simulink model "flexcan_can_fd_master_s32k14"  (R2017a)
settings: Solver=FixedStepDiscrete  StartTime=0.0  StopTime=10.0  FixedStep=0.1  RelTol=1e-3  EnableMultiTasking=on
InitFcn:
  | mbd_s32k14_consistency_checks(bdroot(gcs));
undefined symbols (not defined in the file): B8, C7, D1, D2, G2, PTC6, PTC7, PTD16, PTE4, PTE5, raw_temp
libraries: mbd_s32k14_ec_toolbox x10, etargetslib x1, simulink x1
Description:
  | This model tests FlexCAN communication using CAN with Flexible Data-Rate.
  | The FlexCAN Master sends on each step a message with ID 0x3FF to the slave.
  | On each Tx Complete event Blue LED (PTD0) is toggled.
  | 
  | HW prerequisite:
  | - S32K144EVB-Q100
  | - Make sure that J107 has pin 1 and 2 connected and external power supply is provieded through J16.
  | 
  | Validation:
  | - The CAN Baudrate is set to 500 Kb/s
  | - Any CAN analizer (USB to CAN device) can be used to observe CAN traffic via board CAN port J13.
settings Model: Creator=agrigorev  LastModifiedBy=Siddharth
settings DataIOCC: ExternalInput=off  InitialState=off  LimitDataPoints=on  SaveFormat=Array  SaveOutput=off  SignalLogging=off  SaveTime=off
settings OptimizationCC: DefaultParameterBehavior=Inlined  PassReuseOutputArgsAs=Individual arguments
settings DebuggingCC: UnderspecifiedInitializationDetection=Classic  MergeDetectMultiDrivingBlocksExec=none  SolverPrmCheckMsg=warning  InheritedTsInSrcMsg=none  SingleTaskRateTransMsg=error  ParameterTunabilityLossMsg=error  UnconnectedInputMsg=error  UnconnectedOutputMsg=error  UnconnectedLineMsg=error  AllowSymbolicDim=off  UnknownTsInhSupMsg=error  StateNameClashWarn=warning  SFUnexpectedBacktrackingDiag=warning  SFNoUnconditionalDefaultTransitionDiag=warning  SFExecutionAtInitializationDiag=none
settings HardwareCC: ProdBitPerPointer=32  ProdBitPerSizeT=32  ProdBitPerPtrDiffT=32  ProdLargestAtomicInteger=Long  ProdLargestAtomicFloat=Double  ProdWordSize=32  ProdHWDeviceType=ARM Compatible->ARM Cortex
settings ModelReferenceCC: PropagateSignalLabelsOutOfModel=off
settings SFSimCC: MATLABDynamicMemAlloc=off
settings RTWCC: SystemTargetFile=mbd_s32k14.tlc  MakeCommand=mbd_s32k14_make_rtw COPY_MDLREF_INCLUDES=0  TemplateMakefile=mbd_s32k14.tmf  Description=Model Based Design Toolbox S32K14x Code Generation Target  GenerateReport=on  IncludeHyperlinkInReport=on  LaunchReport=on  GenerateTraceInfo=on  GenerateTraceReport=on  GenerateTraceReportSl=on  GenerateTraceReportSf=on  GenerateTraceReportEml=on
settings CodeAppCC: ForceParamTrailComments=on  IgnoreCustomStorageClasses=off  OperatorAnnotations=on  SimulinkDataObjDesc=on  SFDataObjDesc=on  MATLABFcnDesc=on  InsertBlockDesc=on  MATLABSourceComments=on
settings STFCustomTargetCC: MultiwordLength=256  CombineOutputUpdateFcns=on  ERTCustomFileBanners=on  SupportContinuousTime=off  SupportNonInlinedSFcns=off  RemoveResetFunc=on  MATLABClassNameForMDSCustomization=Simulink.SoftwareTarget.ERTCustomization  GRTInterface=off  SystemTargetFile=mbd_s32k14.tlc
settings ERTTargetCC: ParMdlRefBuildCompliant=off  CompOptLevelCompliant=off  ConcurrentExecutionCompliant=off  ERTFirstTimeCompliant=off  ModelStepFunctionPrototypeControlCompliant=off  CPPClassGenCompliant=off  UseToolchainInfoCompliant=off  InlinedParameterPlacement=NonHierarchical  ERTCustomFileTemplate=example_file_process.tlc
settings ConfigComp: CovMetricSettings=dw  CovHtmlReporting=on  CovSaveCumulativeToWorkspaceVar=on  CovSaveSingleToWorkspaceVar=on  CovExternalEMLEnable=off

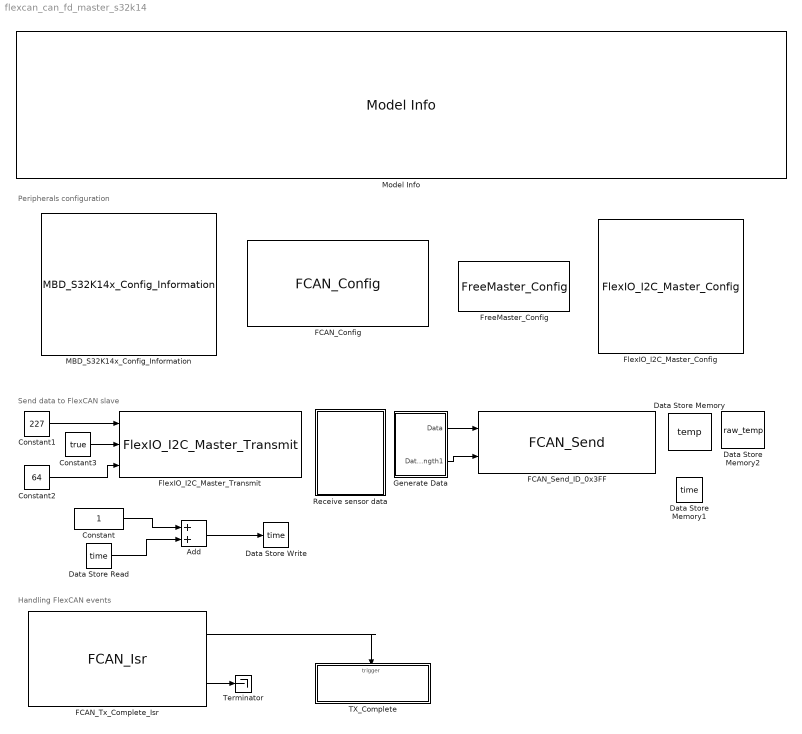
== system flexcan_can_fd_master_s32k14 ==
  note: Peripherals configuration
  note: Handling FlexCAN events
  note: Send data to FlexCAN slave
  Add : Sum  AccumDataTypeStr=uint32  OutDataTypeStr=uint32
  Constant : Constant  OutDataTypeStr=uint32
  Constant1 : Constant  Value=227  OutDataTypeStr=uint8
  Constant2 : Constant  Value=64  OutDataTypeStr=uint8
  Constant3 : Constant  Value=true
  Data Store Memory : DataStoreMemory  DataStoreName=temp  ReadBeforeWriteMsg=warning  WriteAfterWriteMsg=warning  WriteAfterReadMsg=warning  ShowAdditionalParam=off
  Data Store Memory1 : DataStoreMemory  DataStoreName=time  ReadBeforeWriteMsg=warning  WriteAfterWriteMsg=warning  WriteAfterReadMsg=warning  ShowAdditionalParam=off  OutDataTypeStr=uint32
  Data Store Memory2 : DataStoreMemory  DataStoreName=raw_temp  ReadBeforeWriteMsg=warning  WriteAfterWriteMsg=warning  WriteAfterReadMsg=warning  InitialValue=[0 0]  ShowAdditionalParam=off  OutDataTypeStr=uint8  Dimensions=2
  Data Store Read : DataStoreRead  DataStoreName=time
  Data Store Write : DataStoreWrite  DataStoreName=time
  FCAN_Config : mbd_s32k14_ec_toolbox/S32K14x/Communication Blocks/Flex CAN Blocks/FCAN_Config  Priority=1  can_instance=0  can_mode=Normal mode  can_max_num_mb=16  can_rx=PTE4 : [9] : [6] : [D1]  can_tx=PTE5 : [8] : [5] : [D2]  show_adv_opts=on  can_clk_src=Peripheral clock  can_presdiv=9  can_rjw=0  can_pseg1=3  can_pseg2=3  can_propseg=6  can_cbt_presdiv=9  can_cbt_rjw=0  can_cbt_pseg1=3  can_cbt_pseg2=3  can_cbt_propseg=6  can_fd_enable=on  can_payload=8  can_rxfifo_enable=off  can_fifo_id_filter_extended=off  can_fifo_id_filter_remote=off  can_num_id_filters=8  can_fifo_id_format=A  can_fifo_id_filter={'0x0', '0x0', '0x0', '0x0', '0x0', '0x0', '0x0', '0x0'}  can_pn_enable=off  can_wakeup_match=off  can_wakeup_timeout=off  can_timeout_en=off  can_match_timeout=1  can_multiple_matches_en=off  can_num_matches=1  can_idfilter_extendedid=off  can_idfilter_remoteframe=off  can_idfilter_type=Match exact  can_idfilter_id1=0  can_idfilter_id2=0  can_payloadfilter_enable=off  can_payloadfilter_dlclow=0  can_payloadfilter_dlchigh=0  can_payloadfilter_type=Match exact  can_payloadfilter_payload1_b0=0  can_payloadfilter_payload1_b1=0  can_payloadfilter_payload1_b2=0  can_payloadfilter_payload1_b3=0  can_payloadfilter_payload1_b4=0  can_payloadfilter_payload1_b5=0  can_payloadfilter_payload1_b6=0  can_payloadfilter_payload1_b7=0  can_payloadfilter_payload2_b0=0  can_payloadfilter_payload2_b1=0  can_payloadfilter_payload2_b2=0  can_payloadfilter_payload2_b3=0  can_payloadfilter_payload2_b4=0  can_payloadfilter_payload2_b5=0  can_payloadfilter_payload2_b6=0  can_payloadfilter_payload2_b7=0
  FCAN_Send_ID_0x3FF : mbd_s32k14_ec_toolbox/S32K14x/Communication Blocks/Flex CAN Blocks/FCAN_Send  Priority=2  can_instance=0  can_mode=Non-blocking  can_timeout_ms=0  can_mb_idx=15  can_extended_id=off  can_is_remote=off  can_id=3FF  show_adv_opts=on  can_fd_enable=on  can_enable_brs=off  can_fd_padding=0
  FCAN_Tx_Complete_Isr : mbd_s32k14_ec_toolbox/S32K14x/Communication Blocks/Flex CAN Blocks/FCAN_Isr  can_instance=0  can_event=Tx Complete
  "FlexIO_I2C_Master_Config " : mbd_s32k14_ec_toolbox/S32K14x/Communication Blocks/FlexIO Blocks /FlexIO I2C Blocks/FlexIO_I2C_Master_Config   InstanceNumber=0  DriverType=Polling  BaudRate=400000  SDA_pin=[PTD0] FXIO_D0  SCL_pin=[PTD1] FXIO_D1
  FlexIO_I2C_Master_Transmit : mbd_s32k14_ec_toolbox/S32K14x/Communication Blocks/FlexIO Blocks /FlexIO I2C Blocks/FlexIO_I2C_Master_Transmit  InstanceNumber=0  Timeout=10
  FreeMaster_Config : mbd_s32k14_ec_toolbox/S32K14x/Utility Blocks/FreeMaster_Config  interface=UART1  baudrate=57600  rxd=PTC6 : [81] : [52] : [C7]  txd=PTC7 : [80] : [51] : [B8]  mode=Poll-driven  isr_prio=15  show_adv_opts=off  use_scope=on  max_scope_vars=8  use_recorder=on  max_rec_vars=8  rec_buff_size=1024  rec_timebase=0 seconds  comm_buffer_size_auto=on  comm_buffer_size=255  comm_rqueue_size_default=on  comm_rqueue_size=32
  Generate Data : Subsystem
  MBD_S32K14x_Config_Information : mbd_s32k14_ec_toolbox/S32K14x/MBD_S32K14x_Config_Information  disp_str=|  config_params=[]
      | Target : S32K144-64KB_SRAM
      | Package : 100-pin
      | System clock : 80 MHz
      | XTAL clock : External 8 MHz
      | Compiler : GCC
      | Target Type : FLASH
      | Download Code after build : (OpenSDA: F)
      | Step Tick Interrupt Priority : 15
  Model Info : simulink/Model-Wide Utilities/Model Info  Frame=off  DisplayStringWithTags=|  HorizontalTextAlignment=Left  LeftAlignmentValue=0.02  SourceBlockDiagram=flexcan_can_fd_master_s32k14  TagMaxNumber=20
      | Model Name: %<ModelName>
      | 
      | Description: %<Description>
  Receive sensor data : Subsystem
  TX_Complete : Subsystem  TreatAsAtomicUnit=on
      settings: RTWSystemCode=Nonreusable function
  Terminator : Terminator
  wires:
  FCAN_Tx_Complete_Isr/2 -> Terminator/1
  Generate Data/2(Data Length1) -> FCAN_Send_ID_0x3FF/2
  Generate Data/1(Data) -> FCAN_Send_ID_0x3FF/1
  FCAN_Tx_Complete_Isr/1 -> TX_Complete/Trigger
  Constant2/1 -> FlexIO_I2C_Master_Transmit/3
  Constant1/1 -> FlexIO_I2C_Master_Transmit/1
  Constant3/1 -> FlexIO_I2C_Master_Transmit/2
  Constant/1 -> Add/1
  Data Store Read/1 -> Add/2
  Add/1 -> Data Store Write/1

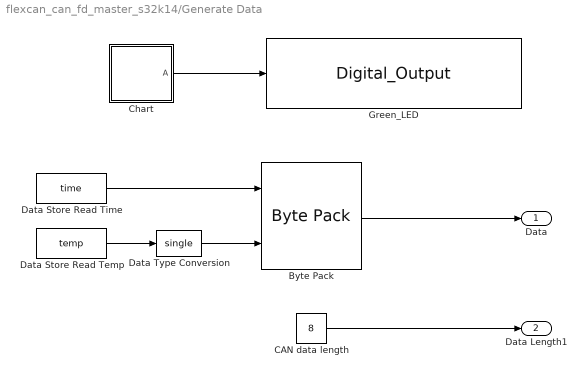
== system flexcan_can_fd_master_s32k14/Generate Data ==
  Byte Pack : etargetslib/Byte Pack  datatypes={'uint32','single'}  byteAlign=1
  CAN data length : Constant  Value=8  OutDataTypeStr=uint8
  Chart : Stateflow chart  TreatAsAtomicUnit=on
  Data Store Read Temp : DataStoreRead  DataStoreName=temp
  Data Store Read Time : DataStoreRead  DataStoreName=time
  Data Type Conversion : DataTypeConversion  OutDataTypeStr=single
  Green_LED : mbd_s32k14_ec_toolbox/S32K14x/Peripheral Interface Blocks/Digital_Output  gpio_pin=PTD16 : [21] : [14] : [G2]  port=D  pin=16  drive_strength=Low  slew_rate=Fast
  Data : Outport
  Data Length1 : Outport  Port=2
  wires:
  Chart/1(" A") -> Green_LED/1
  Data Store Read Time/1 -> Byte Pack/1
  CAN data length/1 -> Data Length1/1
  Byte Pack/1 -> Data/1
  Data Type Conversion/1 -> Byte Pack/2
  Data Store Read Temp/1 -> Data Type Conversion/1

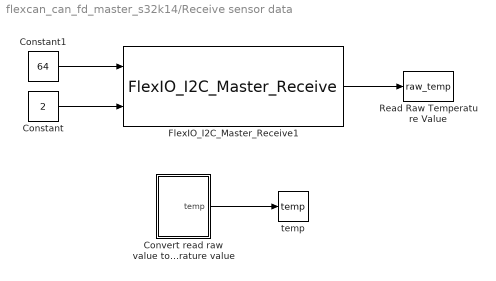
== system flexcan_can_fd_master_s32k14/Receive sensor data ==
  Constant : Constant  Value=2  OutDataTypeStr=uint32
  Constant1 : Constant  Value=64  OutDataTypeStr=uint8
  Convert read raw value to temperature value : Subsystem
  FlexIO_I2C_Master_Receive1 : mbd_s32k14_ec_toolbox/S32K14x/Communication Blocks/FlexIO Blocks /FlexIO I2C Blocks/FlexIO_I2C_Master_Receive  InstanceNumber=0  Timeout=10
  Read Raw Temperature Value : DataStoreWrite  DataStoreName=raw_temp
  temp : DataStoreWrite  DataStoreName=temp
  wires:
  Convert read raw value to temperature value/1(temp) -> temp/1
  Constant1/1 -> FlexIO_I2C_Master_Receive1/1
  Constant/1 -> FlexIO_I2C_Master_Receive1/2
  FlexIO_I2C_Master_Receive1/1 -> Read Raw Temperature Value/1

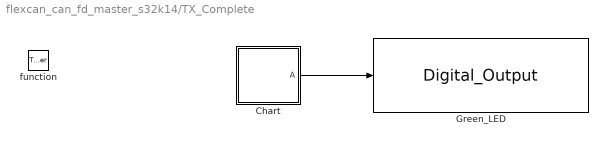
== system flexcan_can_fd_master_s32k14/TX_Complete ==
  function : TriggerPort  TriggerType=function-call  VariantControl=Variant
  Chart : Stateflow chart  TreatAsAtomicUnit=on
  Green_LED : mbd_s32k14_ec_toolbox/S32K14x/Peripheral Interface Blocks/Digital_Output  gpio_pin=PTD16 : [21] : [14] : [G2]  port=D  pin=16  drive_strength=Low  slew_rate=Fast
  wires:
  Chart/1(" A") -> Green_LED/1

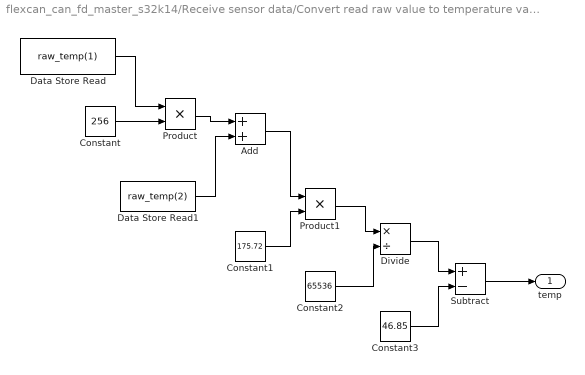
== system flexcan_can_fd_master_s32k14/Receive sensor data/Convert read raw value to temperature value ==
  Add : Sum
  Constant : Constant  Value=256
  Constant1 : Constant  Value=175.72
  Constant2 : Constant  Value=65536
  Constant3 : Constant  Value=46.85
  Data Store Read : DataStoreRead  DataStoreName=raw_temp  DataStoreElements=raw_temp(1)
  Data Store Read1 : DataStoreRead  DataStoreName=raw_temp  DataStoreElements=raw_temp(2)
  Divide : Product  Inputs=*/
  Product : Product
  Product1 : Product
  Subtract : Sum  Inputs=+-
  temp : Outport
  wires:
  Constant/1 -> Product/2
  Product/1 -> Add/1
  Data Store Read1/1 -> Add/2
  Add/1 -> Product1/1
  Constant1/1 -> Product1/2
  Product1/1 -> Divide/1
  Constant2/1 -> Divide/2
  Divide/1 -> Subtract/1
  Constant3/1 -> Subtract/2
  Subtract/1 -> temp/1
  Data Store Read/1 -> Product/1

== stateflow chart flexcan_can_fd_master_s32k14/Generate Data/Chart ==
  state A
  state A1
  (default) -> A
  A -> A1
  A1 -> A
  data: A output boolean [0..1]

== stateflow chart flexcan_can_fd_master_s32k14/TX_Complete/Chart ==
  state A
  state A1
  (default) -> A
  A -> A1
  A1 -> A
  data: A output boolean [0..1]
